simulink model "oscillateur"  (R2019b)
settings: Solver=ode23t  StartTime=0.0  StopTime=100  RelTol=1e-3
InitFcn:
  | b = 0.05;
  | k = 0.3;
  | m = 0.5;
  | F = 20;
settings Model: Creator=ivanl  LastModifiedBy=ivanl

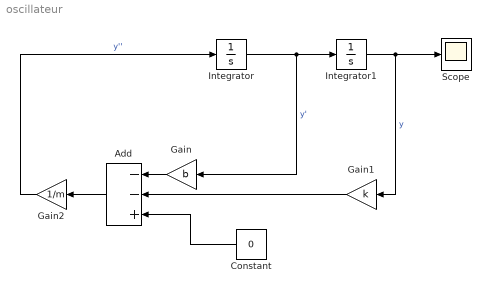
== system oscillateur ==
  Add : Sum  Inputs=--+
  Constant : Constant  Value=0
  Gain : Gain  Gain=b
  Gain1 : Gain  Gain=k
  Gain2 : Gain  Gain=1/m
  Integrator : Integrator
  Integrator1 : Integrator  InitialCondition=1
  Scope : Scope
  wires:
  Integrator/1 -> Gain/1, Integrator1/1  "y'"
  Gain2/1 -> Integrator/1  "y''"
  Gain/1 -> Add/1
  Gain1/1 -> Add/2
  Integrator1/1 -> Gain1/1, Scope/1  "y"
  Add/1 -> Gain2/1
  Constant/1 -> Add/3
